simulink model "PassengerCar"  (R2019b)
settings: Solver=ode1  StartTime=0  StopTime=25  FixedStep=1.0000000000000000e-003  RelTol=1e-3
InitFcn:
  | sampleTime = str2double(get_param(bdroot, 'FixedStep'));
undefined symbols (not defined in the file or in its folder): AccPedalPos, BrakePedalPos, BrakeSwitch, DiscIntNeverNeededParam, DYNA4, EngSpd, IgnitionSwitch, InitialGear, InitialSpeed, IntendedEngTrq, LeftIndicator, MainBrakePress, MaxGear, MDL, MinGear, RefAcc, RefLane, RefLatPos, RefPath, RefPathCurv, RefSpd, RefSpdPreview, RefSpdRetrospect, RightIndicator, SteeringWheelAng, SteeringWheelTrq, UserDefinedRefValue, vm_const
libraries: UtilitiesLibrary x31, simulink x18, WheelSystemModules x13, LongitudinalControllerModules x13, LateralControllerModules x7, AnimationBusselectorModules x5, EnvironmentModules x5, BasicEngineControlModules x5, MiscellaneousControlModules x5, Animation3Modules x4, AuxiliariesModules x4, TireModules x4
(part 39 of 39)

== system PassengerCar/VehicleControl/LongitudinalControl/ControlSystems/Longitudinal Controller/Acceleration Control/ComputeBrakePedalPos/no Brake AND Gas ==
  AccPedal : Inport
  BrakePedal : Inport  Port=2
  PedalChangeTime : Inport  Port=3
  Constant3 : Constant  Value=1e-3
  Constant4 : Constant  Value=0
  Data Type Conversion : DataTypeConversion  OutDataTypeStr=double  SaturateOnIntegerOverflow=on  RndMeth=Zero
  Integrator : DiscreteIntegrator  ExternalReset=either  SampleTime=-1  ICPrevOutput=DiscIntNeverNeededParam  ICPrevScaledInput=DiscIntNeverNeededParam
  "Pedal Change Time " : RelationalOperator  RndMeth=Nearest  InputSameDT=on
      settings: AttributesFormatString===> Brake allowed
  Switch : Switch  Threshold=0.5
  no Gas1 : RelationalOperator  Operator=>  RndMeth=Nearest  InputSameDT=on
  ModifiedBrakePedalPos [0-1] : Outport  VectorParamsAs1DForOutWhenUnconnected=off
  wires:
  PedalChangeTime/1 -> "Pedal Change Time "/2
  Constant4/1 -> Switch/3
  BrakePedal/1 -> Switch/1
  Switch/1 -> ModifiedBrakePedalPos [0-1]/1
  Constant3/1 -> no Gas1/1
  Integrator/1 -> "Pedal Change Time "/1
  no Gas1/1 -> Data Type Conversion/1
  AccPedal/1 -> no Gas1/2
  "Pedal Change Time "/1 -> Switch/2
  Data Type Conversion/1 -> Integrator/2, Integrator/1

== system PassengerCar/VehicleControl/LongitudinalControl/ControlSystems/Longitudinal Controller/Speed Control/Load Torque Vehicle/toCompile ==

== system PassengerCar/VehicleControl/LongitudinalControl/ControlSystems/Longitudinal Controller/Speed Control/Preprocessing VehicleInfo/DetectGearChange ==
  note: TransmissionType
      | 0 = none
      | 1 = manual
      | 2 = automatic
  Gear : Inport
  TransmissionType : Inport  Port=2
  Data Type Conversion2 : DataTypeConversion  OutDataTypeStr=double
  Default : Constant  Value=0
  Multiport Switch : MultiPortSwitch  DataPortOrder=Zero-based contiguous  Inputs=4  zeroidx=on
  if gear change : RelationalOperator  Operator=~=  OutDataTypeStr=boolean  RndMeth=Nearest  InputSameDT=on
  if neither selected nor previous gear zero : Logic  AllPortsSameDT=off  OutDataTypeStr=boolean
  if neither selected nor previous gear zero1 : Logic
  previous gear : Memory  InheritSampleTime=on
  GearChangeFlag : Outport  VectorParamsAs1DForOutWhenUnconnected=off
  wires:
  if neither selected nor previous gear zero/1 -> if neither selected nor previous gear zero1/2
  if gear change/1 -> if neither selected nor previous gear zero1/1
  Data Type Conversion2/1 -> GearChangeFlag/1
  Gear/1 -> Multiport Switch/5, Multiport Switch/3, Multiport Switch/4  "selected gear"
  Default/1 -> Multiport Switch/2
  TransmissionType/1 -> Multiport Switch/1
  if neither selected nor previous gear zero1/1 -> Data Type Conversion2/1  "gear change (not from/to neutral)"
  Multiport Switch/1 -> previous gear/1, if neither selected nor previous gear zero/2, if gear change/1  "selected gear"
  previous gear/1 -> if neither selected nor previous gear zero/1, if gear change/2  "previous gear"

== system PassengerCar/VehicleControl/LongitudinalControl/ControlSystems/Longitudinal Controller/Speed Control/Preprocessing VehicleInfo/TractionCtrl ==
  ClutchManual [0_1] : Inport
  GearChangeFlag [0|1] : Inport  Port=2
  Constant : Constant  Value=1e-5
  Data Type Conversion : DataTypeConversion  OutDataTypeStr=double  SaturateOnIntegerOverflow=on  RndMeth=Zero
  Data Type Conversion1 : DataTypeConversion  OutDataTypeStr=boolean  SaturateOnIntegerOverflow=on  RndMeth=Zero
  Data Type Conversion2 : DataTypeConversion  OutDataTypeStr=boolean  SaturateOnIntegerOverflow=on  RndMeth=Zero
  Data Type Conversion3 : DataTypeConversion  OutDataTypeStr=double  SaturateOnIntegerOverflow=on  RndMeth=Zero
  Hit Crossing : HitCross  HitCrossingOffset=0.5  HitCrossingDirection=rising
  Relational Operator : RelationalOperator  Operator=>  RndMeth=Nearest
  S-R Flip-Flop : simulink_extras/Flip Flops/S-R Flip-Flop  initial_condition=0
  Terminator : Terminator
  ASRFlag [0/1] : Outport  VectorParamsAs1DForOutWhenUnconnected=off
  wires:
  GearChangeFlag [0|1]/1 -> Data Type Conversion1/1
  S-R Flip-Flop/1 -> Data Type Conversion/1
  Data Type Conversion/1 -> ASRFlag [0/1]/1
  S-R Flip-Flop/2 -> Terminator/1
  ClutchManual [0_1]/1 -> Relational Operator/1
  Constant/1 -> Relational Operator/2
  Relational Operator/1 -> Data Type Conversion3/1
  Hit Crossing/1 -> Data Type Conversion2/1
  Data Type Conversion1/1 -> S-R Flip-Flop/1
  Data Type Conversion2/1 -> S-R Flip-Flop/2
  Data Type Conversion3/1 -> Hit Crossing/1

== system PassengerCar/VehicleControl/LateralControl/Disabled LateralControl/ControlSystems/Lateral Controller/User-Defined Control/UserDefinedControl/DynaModuleInfo ==

== system PassengerCar/VehicleControl/LongitudinalControl/ControlSystems/Longitudinal Controller/Acceleration Control/ComputeBrakePedalPos/Calculate Brake Pedal/Limiter [0-1] ==
  In : Inport
  Limiter : MinMax  Inputs=2  SaturateOnIntegerOverflow=on  InputSameDT=on
  Limiter1 : MinMax  Function=max  Inputs=2  SaturateOnIntegerOverflow=on  InputSameDT=on
  max. brake pedal position : Constant
  min. brake pedal position : Constant  Value=0
  Out : Outport  VectorParamsAs1DForOutWhenUnconnected=off
  wires:
  max. brake pedal position/1 -> Limiter/2
  Limiter/1 -> Limiter1/1
  min. brake pedal position/1 -> Limiter1/2
  In/1 -> Limiter/1
  Limiter1/1 -> Out/1
